simulink model "model_class_1"  (R2018a)
settings: Solver=VariableStepAuto  StartTime=0.0  StopTime=10.0  RelTol=1e-3
settings Model: Creator=NEW PC  LastModifiedBy=NEW PC

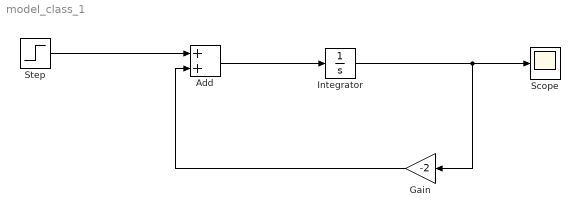
== system model_class_1 ==
  Add : Sum
  Gain : Gain  Gain=-2
  Integrator : Integrator
  Scope : Scope
  Step : Step  After=3  SampleTime=0
  wires:
  Integrator/1 -> Gain/1, Scope/1
  Add/1 -> Integrator/1
  Gain/1 -> Add/2
  Step/1 -> Add/1
